simulink model "cw5_simulink"  (R2025b)
settings: Solver=VariableStepAuto  StartTime=0.0  StopTime=20  RelTol=1e-3
values from neighbouring files (symbols this model uses):
  h = 42    [cw5_samolot_dane.m]
  k1 = 54.7*1000    (= 54700)    [cw5_samolot_dane.m]
  k2 = 303.6*1000    (= 303600)    [cw5_samolot_dane.m]
  m1 = 14000    [cw5_samolot_dane.m]
  m2 = 450.28    [cw5_samolot_dane.m]
  m3 = 200    [cw5_samolot_dane.m]
  v_0 = 67    [cw5_samolot_dane.m]
settings Model: Creator=student  LastModifiedBy=P

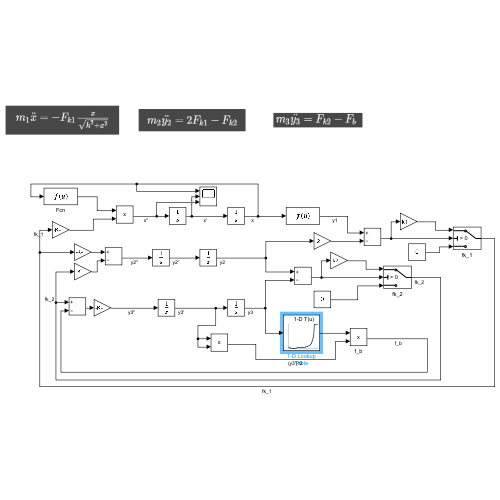
[thumbnail: Simulink's stored preview of the top-level diagram]
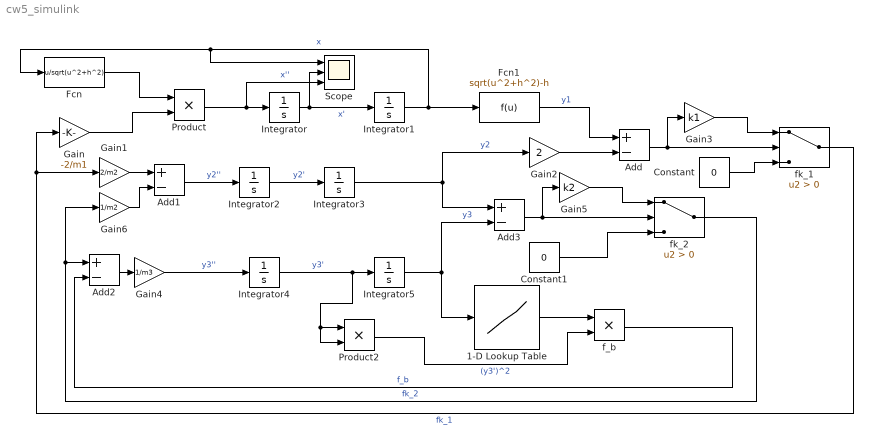
== system cw5_simulink ==
  1-D Lookup Table : Lookup_n-D  NumberOfTableDimensions=1  BreakpointsForDimension1=[0;10;20;30;40;50;60;70;80;90;94;98;102;104;107;120]  Table=[833;400;160;320;520;520;660;830;1070;1600;2100;2800;4100;5000;9000;9000]  InternalRulePriority=Speed  RndMeth=Simplest
  Add{,1..3} (4 alike) : Sum  Inputs=+-
  Constant : Constant  Value=0
  Constant1 : Constant  Value=0
  Fcn : Fcn  Expr=u/sqrt(u^2+h^2)
  Fcn1 : Fcn  Expr=sqrt(u^2+h^2)-h
  Gain : Gain  Gain=-2/m1
  Gain1 : Gain  Gain=2/m2
  Gain2 : Gain  Gain=2
  Gain3 : Gain  Gain=k1
  Gain4 : Gain  Gain=1/m3
  Gain5 : Gain  Gain=k2
  Gain6 : Gain  Gain=1/m2
  Integrator : Integrator  InitialCondition=v_0
  Integrator{1..5} (5 alike) : Integrator
  Product : Product
  Product2 : Product
  Scope : Scope  NumInputPorts=3
      settings: ActiveDisplayYMinimum=-33.02709898001671  ActiveDisplayYMaximum=297.24389082015045
  f_b : Product
  fk_1 : Switch  Criteria=u2 > Threshold  SaturateOnIntegerOverflow=off  InputSameDT=off
  fk_2 : Switch  Criteria=u2 > Threshold  SaturateOnIntegerOverflow=off  InputSameDT=off
  wires:
  Fcn/1 -> Product/1
  Gain/1 -> Product/2
  Product/1 -> Scope/3, Integrator/1  "x''"
  Integrator/1 -> Scope/2, Integrator1/1  "x'"
  Integrator1/1 -> Fcn1/1, Scope/1, Fcn/1  "x"
  fk_1/1 -> Gain/1, Gain1/1  "fk_1"
  Gain2/1 -> Add/2
  Add/1 -> fk_1/2, Gain3/1
  Gain3/1 -> fk_1/1
  Constant/1 -> fk_1/3
  Fcn1/1 -> Add/1  "y1"
  Gain1/1 -> Add1/1
  Add1/1 -> Integrator2/1  "y2''"
  Integrator2/1 -> Integrator3/1  "y2'"
  Integrator3/1 -> Gain2/1, Add3/1  "y2"
  Add2/1 -> Gain4/1
  Integrator4/1 -> Product2/2, Product2/1, Integrator5/1  "y3'"
  Integrator5/1 -> 1-D Lookup Table/1, Add3/2  "y3"
  1-D Lookup Table/1 -> f_b/1
  Product2/1 -> f_b/2  "(y3')^2"
  f_b/1 -> Add2/2  "f_b"
  Constant1/1 -> fk_2/3
  Gain5/1 -> fk_2/1
  Add3/1 -> fk_2/2, Gain5/1
  fk_2/1 -> Gain6/1, Add2/1  "fk_2"
  Gain4/1 -> Integrator4/1  "y3''"
  Gain6/1 -> Add1/2
